simulink model "SwitchingCircuit"  (R2022b)
settings: Solver=VariableStepAuto  StartTime=0.0  StopTime=10.0  RelTol=1e-3
libraries: ee_lib x5, fl_lib x4
settings Model: Creator=mrrobot  LastModifiedBy=mrrobot

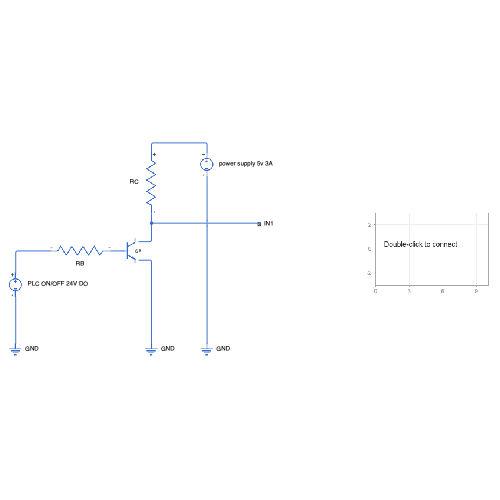
[thumbnail: Simulink's stored preview of the top-level diagram]
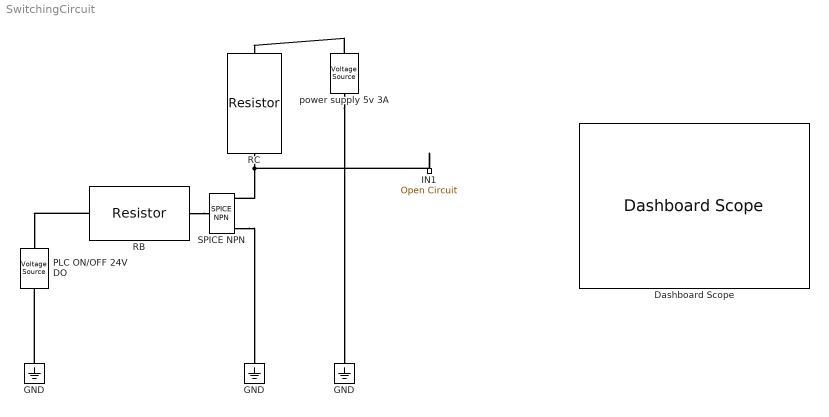
== system SwitchingCircuit ==
  Dashboard Scope : DashboardScope
  GND : fl_lib/Electrical/Electrical Elements/Electrical Reference
  "GND " : fl_lib/Electrical/Electrical Elements/Electrical Reference
  "GND  " : fl_lib/Electrical/Electrical Elements/Electrical Reference
  IN1 : fl_lib/Electrical/Electrical Elements/Open Circuit  v_specify=off  v_priority=None  v=0 V  v_nominal_specify=off  v_nominal_unit=V  v_nominal_value=1
      settings: LibrarySourceBlock=|
      | ee_lib/Connectors &
      | References/Open Circuit
  PLC ON/OFF 24V DO : ee_lib/Sources/Voltage Source  dc_voltage=24 V  ac_voltage=0 V  ac_shift=0 rad  ac_frequency=60 Hz  noise_mode=ee.enum.sources.noise.Disabled  PSD=0 V^2/Hz  sample_time=1e-3 s  repeatability=ee.enum.sources.repeatability.NotRepeatable  user_seed=0  auto_seed=3922919431  i_specify=off  i_priority=None  i=0 A  i_nominal_specify=off  i_nominal_unit=A  i_nominal_value=1  v_specify=off  v_priority=None  v=0 V  v_nominal_specify=off  v_nominal_unit=V  v_nominal_value=1
  RB : ee_lib/Passive/Resistor  R=1 Ohm  enable_R_tol=0  R_tol=5  tol_distribution=1  nSigma=4  enable_operating_limits=0  operating_limit_action=2  max_working_voltage=100 V  power_rating=1 W  enable_faults=0  fault_action=1  R_faulted=inf Ohm  enable_temporal_fault=0  t_fault=1 s  enable_behavioral_fault=0  max_permissible_current=1 A  t_fail_on_current=1 s  noise_mode=0  sample_time=1e-3 s  repeatability=1  auto_seed=3890346746  user_seed=0  Tdevice=25 degC  power_derating_T1=70 degC  power_derating_T2=155 degC  operating_temperature_range_vec=[-50, 150] degC  alpha=3.93e-3 1/K  Tmeas=25 degC  thermal_mass=100 J/K  temperature_specify=off  temperature_priority=High  temperature=298.15 K  temperature_nominal_specify=off  temperature_nominal_unit=K  temperature_nominal_value=1
  RC : ee_lib/Passive/Resistor  R=1 Ohm  enable_R_tol=0  R_tol=5  tol_distribution=1  nSigma=4  enable_operating_limits=0  operating_limit_action=2  max_working_voltage=100 V  power_rating=1 W  enable_faults=0  fault_action=1  R_faulted=inf Ohm  enable_temporal_fault=0  t_fault=1 s  enable_behavioral_fault=0  max_permissible_current=1 A  t_fail_on_current=1 s  noise_mode=0  sample_time=1e-3 s  repeatability=1  auto_seed=3499211588  user_seed=0  Tdevice=25 degC  power_derating_T1=70 degC  power_derating_T2=155 degC  operating_temperature_range_vec=[-50, 150] degC  alpha=3.93e-3 1/K  Tmeas=25 degC  thermal_mass=100 J/K  temperature_specify=off  temperature_priority=High  temperature=298.15 K  temperature_nominal_specify=off  temperature_nominal_unit=K  temperature_nominal_value=1
  SPICE NPN : ee_lib/Additional Components/SPICE Semiconductors/SPICE NPN  AREA=1.0 m^2  SCALE=1  IS=1.0e-16 A/m^2  BF=100.0  NF=1  VAF=Inf V  IKF=Inf A/m^2  ISE=0 A/m^2  NE=1.5  BR=1  NR=1  VAR=Inf V  IKR=Inf A/m^2  ISC=0 A/m^2  NC=2  RB=1 Ohm*m^2  IRB=Inf A/m^2  RBM=0 Ohm*m^2  RE=1e-4 Ohm*m^2  RC=0.01 Ohm*m^2  C_param=1  FC=0.5  IC_given=1  ICVBE=0 V  ICVCE=0 V  CJE=0 F/m^2  VJE=0.75 V  MJE=0.33  TF=0 s  XTF=0  VTF=Inf V  ITF=0 A/m^2  CJC=0 F/m^2  VJC=0.75 V  MJC=0.33  XCJC=1  TR=0 s  CJS=0 F/m^2  VJS=0.75 V  MJS=0  T_param=1  XTB=0  EG=1.11 eV  XTI=3  TFIXED=300.15 K  TMEAS=300.15 K  TOFFSET=0 K
      settings: InternalSimscapePortConfiguration="{\"Bottom\":[],\"Left\":[{\"id\":\"bx\",\"label\":\"\",\"type\":\"foundation.electrical.electrical\"}],\"Right\":[{\"id\":\"cx\",\"label\":\"\",\"type\":\"foundation.electrical.electrical\"},{\"id\":\"sx\",\"label\":\"s\",\"type\":\"foundation.electrical.electrical\"},{\"id\":\"ex\",\"label\":\"\",\"type\":\"foundation.electrical.electrical\"}],\"Top\":[]}"
  power supply 5v 3A : ee_lib/Sources/Voltage Source  dc_voltage=5 V  ac_voltage=0 V  ac_shift=0 rad  ac_frequency=60 Hz  noise_mode=ee.enum.sources.noise.Disabled  PSD=0 V^2/Hz  sample_time=1e-3 s  repeatability=ee.enum.sources.repeatability.NotRepeatable  user_seed=0  auto_seed=545404223  i_specify=off  i_priority=None  i=0 A  i_nominal_specify=off  i_nominal_unit=A  i_nominal_value=1  v_specify=off  v_priority=None  v=0 V  v_nominal_specify=off  v_nominal_unit=V  v_nominal_value=1
  connections:
  power supply 5v 3A/LConn1 -- RC/LConn1
  RB/RConn1 -- SPICE NPN/LConn1
  power supply 5v 3A/RConn1 -- GND/LConn1
  SPICE NPN/RConn3 -- "GND  "/LConn1
  "GND "/LConn1 -- PLC ON/OFF 24V DO/RConn1
  IN1/LConn1 -- RC/RConn1 -- SPICE NPN/RConn1
  RB/LConn1 -- PLC ON/OFF 24V DO/LConn1
